simulink model "Laplace"  (R2019a)
settings: Solver=VariableStepAuto  StartTime=0.0  StopTime=10.0  RelTol=1e-3
settings Model: Creator=Yuval  LastModifiedBy=Yuval

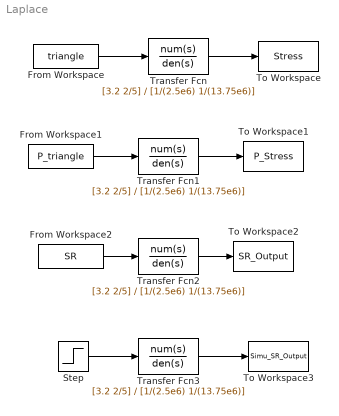
== system Laplace ==
  From Workspace : FromWorkspace  VariableName=triangle  SampleTime=0
  From Workspace1 : FromWorkspace  VariableName=P_triangle  SampleTime=0
  From Workspace2 : FromWorkspace  VariableName=SR  SampleTime=0
  Step : Step  Time=0  After=15/80  SampleTime=0
  To Workspace : ToWorkspace  VariableName=Stress  SaveFormat=Timeseries  SampleTime=-1
  To Workspace1 : ToWorkspace  VariableName=P_Stress  SaveFormat=Timeseries  SampleTime=-1
  To Workspace2 : ToWorkspace  VariableName=SR_Output  SaveFormat=Timeseries  SampleTime=-1
  To Workspace3 : ToWorkspace  VariableName=Simu_SR_Output  SaveFormat=Timeseries  SampleTime=-1
  Transfer Fcn{,1..3} (4 alike) : TransferFcn  Numerator=[3.2 2/5]  Denominator=[1/(2.5e6) 1/(13.75e6)]
  wires:
  Transfer Fcn/1 -> To Workspace/1
  Transfer Fcn1/1 -> To Workspace1/1
  From Workspace1/1 -> Transfer Fcn1/1
  From Workspace2/1 -> Transfer Fcn2/1
  Transfer Fcn2/1 -> To Workspace2/1
  Step/1 -> Transfer Fcn3/1
  Transfer Fcn3/1 -> To Workspace3/1
  From Workspace/1 -> Transfer Fcn/1
